simulink model "ysw11_20"  (R2014a)
settings: Solver=ode45  StartTime=0.0  StopTime=10.0  RelTol=1e-3
libraries: commdigbbndpm3 x1
settings Model: Creator=ii  LastModifiedBy=ii
settings SolverCC: ZeroCrossAlgorithm=Adaptive
settings DebuggingCC: UnderspecifiedInitializationDetection=Classic

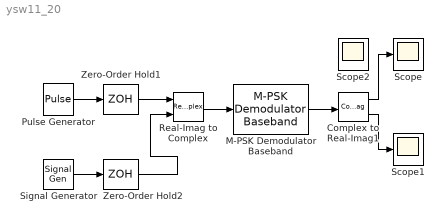
== system ysw11_20 ==
  Complex to Real-Imag1 : ComplexToRealImag
  M-PSK Demodulator Baseband : commdigbbndpm3/M-PSK Demodulator Baseband  M=8  Ph=pi/8  Dec=Gray  Mapping=[0:7]  OutType=Integer  DecType=Hard decision  VarSource=Dialog  Variance=1  outDtype1=Inherit via internal rule  outDtype2=Inherit via internal rule  derotateFactorWordLen=16
  Pulse Generator : DiscretePulseGenerator  PulseType=Time based  Amplitude=300  Period=10  PulseWidth=5
  Real-Imag to Complex : RealImagToComplex
  Scope : Scope
  Scope1 : Scope
  Scope2 : Scope
      settings: SaveName=ScopeData2
  Signal Generator : SignalGenerator  Amplitude=100  Frequency=1000  Units=rad/sec
  Zero-Order Hold1 : ZeroOrderHold
  Zero-Order Hold2 : ZeroOrderHold
  wires:
  Complex to Real-Imag1/1 -> Scope/1
  Complex to Real-Imag1/2 -> Scope1/1
  Zero-Order Hold1/1 -> Real-Imag to Complex/1
  Pulse Generator/1 -> Zero-Order Hold1/1
  Signal Generator/1 -> Zero-Order Hold2/1
  Zero-Order Hold2/1 -> Real-Imag to Complex/2
  Real-Imag to Complex/1 -> M-PSK Demodulator Baseband/1
  M-PSK Demodulator Baseband/1 -> Complex to Real-Imag1/1
